simulink model "pfc"  (R2025b)
settings: Solver=VariableStepAuto  StartTime=0.0  StopTime=5  RelTol=1e-3
undefined symbols (not defined in the file): alpha, DiscIntNeverNeededParam, Ilimit, Izcd, K_Ton_max, Kff, Ki, Kp, Ncycle_min, Ton_max, Ton_min, Ton_startup_max, Ts_ctrl, Ts_v, Tstart, Vin_ff_max, Vin_ff_min, Vovp, Vref
libraries: fl_lib x29, nesl_utility x22, simulink x16, ee_lib x7, eeGeneralControl x4
settings Model: Creator=nickj  LastModifiedBy=nickj
settings DataIOCC: SignalLogging=off  DSMLogging=off  ReturnWorkspaceOutputs=off  LoggingIntervals=[4.8, 5]

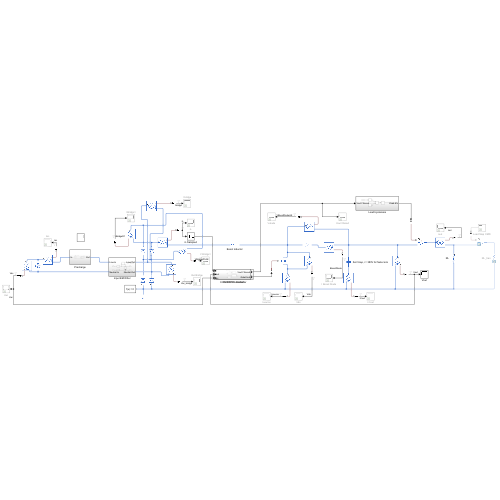
[thumbnail: Simulink's stored preview of the top-level diagram]
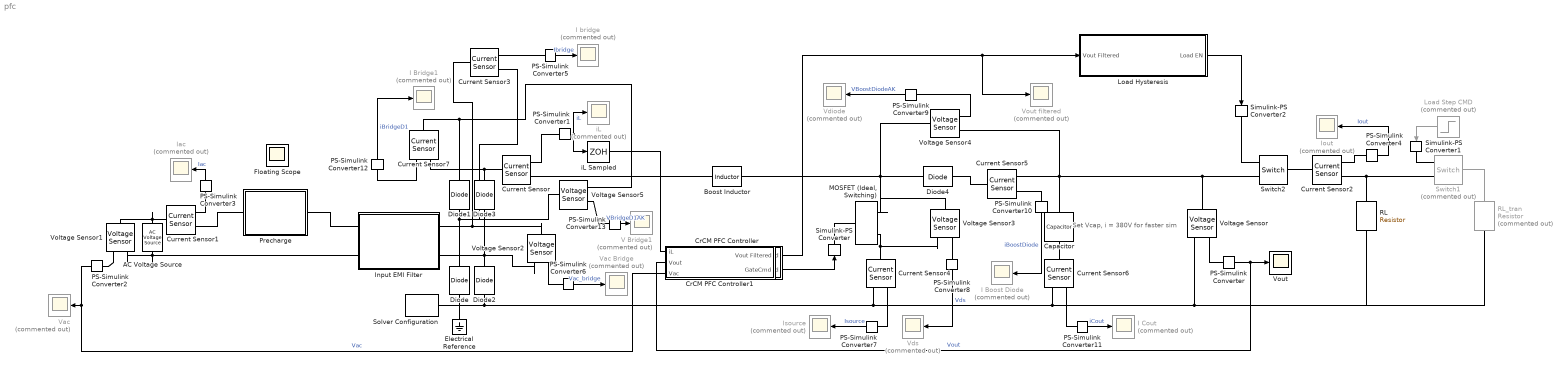
== system pfc ==
  note: Set Vcap, i = 380V for faster sim
  AC Voltage Source : fl_lib/Electrical/Electrical Sources/AC Voltage Source  amp=240*sqrt(2) V  shift=0 deg  frequency=60 Hz
  Boost Inductor : ee_lib/Passive/Inductor  l=270 uH  enable_L_tol=ee.enum.toleranceApplication.none  L_tol=20  tol_distribution=ee.enum.toleranceDistribution.uniform  nSigma=4  r=0.1 Ohm  g=1e-9 1/Ohm  enable_operating_limits=ee.enum.enable.no  operating_limit_action=ee.enum.passive.reportOpLim.warn  max_working_current=1 A  power_rating=1 W  i_L_specify=off  i_L_priority=High  i_L=0 A  i_L_nominal_specify=off  i_L_nominal_value=1  i_L_nominal_unit=A
  Capacitor : ee_lib/Passive/Capacitor  cap_option=ee.enum.passive.capacitor.capOption.const  c=220 uF  Cvec=[1e-05, 1e-06] F  Vvec=[0, 10] V  CV_table_symmetry=ee.enum.passive.capacitor.tableSymmetry.yes  f_vec=[1, 10] kHz  DFext_vec=[.8, 1.2]  enable_C_tol=ee.enum.toleranceApplication.none  averaging_period=0 s  C_tol=5  tol_distribution=ee.enum.toleranceDistribution.uniform  nSigma=4  r=0.3 Ohm  g=0 1/Ohm  enable_operating_limits=ee.enum.enable.no  operating_limit_action=ee.enum.passive.reportOpLim.warn  max_working_voltage_range=[-25, 25] V  power_rating=1 W  maxTemperature=85 degC  thermalEnable=false  thermalMass=1 J/K  i_specify=off  i_priority=None  i=0 A  i_nominal_specify=off  i_nominal_value=1  i_nominal_unit=A  v_specify=off  v_priority=None  v=380 V  v_nominal_specify=off  v_nominal_value=1  v_nominal_unit=V  vc_specify=off  vc_priority=High  vc=380 V  vc_nominal_specify=off  vc_nominal_value=1  vc_nominal_unit=V  T_specify=off  T_priority=None  T=298.15 K  T_nominal_specify=off  T_nominal_value=1  T_nominal_unit=K
  CrCM PFC Controller : Subsystem
  CrCM PFC Controller1 : Subsystem
  Current Sensor{,1..7} (8 alike) : fl_lib/Electrical/Electrical Sensors/Current Sensor
  Diode{,1..4} (5 alike) : fl_lib/Electrical/Electrical Elements/Diode  Vf=0.6 V  Ron=0.3 Ohm  Goff=1e-8 1/Ohm  i_specify=off  i_priority=None  i=0 A  i_nominal_specify=off  i_nominal_value=1  i_nominal_unit=A  v_specify=off  v_priority=None  v=0 V  v_nominal_specify=off  v_nominal_value=1  v_nominal_unit=V
  Electrical Reference : fl_lib/Electrical/Electrical Elements/Electrical Reference
  Floating Scope : Scope
      settings: IsFloating=on  Floating=on  ActiveDisplayString=4  Title=Gate CMD  ActiveDisplayYMinimum=-1.2499999999999998  ActiveDisplayYMaximum=11.25  DataLoggingVariableName=ScopeData33
  I Boost Diode : Scope  Commented=on
      settings: ActiveDisplayYMinimum=-50.843124756105674  ActiveDisplayYMaximum=457.58812280495118  DataLoggingVariableName=ScopeData24
  I Bridge1 : Scope  Commented=on
      settings: ActiveDisplayYMinimum=-7.204509005797358  ActiveDisplayYMaximum=47.078291389116806  DataLoggingVariableName=ScopeData26
  I Cout : Scope  Commented=on
      settings: ActiveDisplayYMinimum=-5.1833261982734609  ActiveDisplayYMaximum=46.649935784461157  DataLoggingVariableName=ScopeData25
  I bridge : Scope  Commented=on
      settings: ActiveDisplayYMinimum=-7.204509005797358  ActiveDisplayYMaximum=47.078291389116806  DataLoggingVariableName=ScopeData7
  Iac : Scope  Commented=on
      settings: ActiveDisplayYMinimum=-2.7208859223508548  ActiveDisplayYMaximum=2.8418563548590066  DataLoggingVariableName=ScopeData4
  Input EMI Filter : Subsystem
  Iout : Scope  Commented=on
      settings: ActiveDisplayYMinimum=-1.2771903163743626E-6  ActiveDisplayYMaximum=1.0183485230584859E-6  DataLoggingVariableName=ScopeData5
  Isource : Scope  Commented=on
      settings: ActiveDisplayYMinimum=-0.14948401946026615  ActiveDisplayYMaximum=1.3453561751423957  DataLoggingVariableName=ScopeData10
  Load Hysteresis : Subsystem
  Load Step CMD : Step  Commented=on  Time=2.5  Before=1  After=0  SampleTime=Ts_v
  "MOSFET (Ideal, Switching)" : ee_lib/Semiconductors & Converters/MOSFET (Ideal, Switching)  port_option=ee.enum.controlport.ps  Rds=0.3 Ohm  Goff=1e-8 1/Ohm  Vth=2 V  diode_param=ee.enum.semiconductors.protectionDiode.nodynamics  diode_Vf=0.8 V  diode_Ron=0.001 Ohm  diode_Goff=1e-5 1/Ohm  diode_C=50e-9 F  diode_iRM=-235 A  diode_iF=300 A  diode_idot=-50 A/us  diode_trr_param=ee.enum.converters.diodeReverseParam.trr_factor  diode_trr_factor=3  diode_trr=15 us  diode_Qrr=1500 s*uA  ids_specify=off  ids_priority=None  ids=0 A  ids_nominal_specify=off  ids_nominal_value=1  ids_nominal_unit=A  vds_specify=off  vds_priority=None  vds=0 V  vds_nominal_specify=off  vds_nominal_value=1  vds_nominal_unit=V  vgs_specify=off  vgs_priority=None  vgs=0 V  vgs_nominal_specify=off  vgs_nominal_value=1  vgs_nominal_unit=V  thermal_loss_option=ee.enum.converters.thermalLossOption.constantvalues  Von_data=[0, 1.8, 3.2, 6, 10, 16; 0, 2, 5.5, 9.5, 15, 25] V  Tj=[298.15, 448.15] K  Iout_data=[0, 20, 40, 60, 80, 100] A  Eon_data=[0, 55.04, 124.57, 235.53, 362.12; 0, 71.25, 161.25, 304.88, 468.75] * 1e-6 J  Eoff_data=[0, 18, 30, 56.1, 76.5; 0, 22.5, 37.5, 70.13, 95.63] * 1e-6 J  Eon_data_3D=[zeros(2, 5, 3)] J  Eoff_data_3D=[zeros(2, 5, 3)] J  Tj_loss=[298.15, 448.15] K  Iout_data_loss=[0, 10, 20, 30, 40] A  tabulateWithVds=false  Vds_loss=[0, 150, 300] V  Eon_scalar=22.86e-3 J  Eoff_scalar=17.14e-3 J  Voff=300 V  Iout_scalar=600 A  useCurrentFromPreviousCycle=false  useVoltageFromPreviousCycle=false  diodeModelType=ee.enum.converters.diodeModelType.pwl  diodeTableType=ee.enum.diode.tableType.IfMat  diode_ReverseIVType=ee.enum.diode.diodeReverseIV.constant  diode_IfMat=[.07, .12, .19, 1.75, 4.24, 7.32, 11.2; .16, .3, .72, 2.14, 4.02, 6.35, 9.12] A  diode_VfMat=[.9, 1.15, 1.25, 1.5, 1.75, 2.17, 2.6, 2.85; .58, .68, .75, 1.1, 1.38, 1.77, 2.27, 2.7] V  diode_TjVec=[25, 125] degC  diode_VfVec=[.5, .7, .9, 1.3, 1.7, 2.1, 2.5] V  diode_IfVec=[.1, .2, .5, 1, 2, 4, 7, 10] A  diode_IrMat=[1e-06, 2e-06, 5e-06, 1e-05, 2.5e-05, 5e-05, .0001; 2e-06, 5e-06, 1e-05, 4e-05, 8e-05, .0002, .0005] A  diode_VrMat=[10, 100, 200, 250, 300, 325, 350; 10, 70, 160, 220, 270, 300, 320] V  diode_VrVec=[10, 20, 40, 50, 70, 80, 100] V  diode_IrVec=[1e-06, 2e-06, 5e-06, 1e-05, 2e-05, 5e-05, .0001] A  diode_Vr=-600 V  diode_Ls=150 nH  diode_Erec=0.03 J  diode_rec_loss_model=ee.enum.diode.reverseRecoveryModel.fixed  diode_ErecVal=0 J  diode_scaleWithIandV=true  diode_ErecMat=zeros(2, 3) J  diode_TjrecVec=[298.15, 398.15] K  diode_IfrecVec=[.1, 1, 10] A  diode_IrecVal=10 A  diode_VrecVal=10 V  diode_tFilter=1 / 1000 / 100 s  separateThermalPortForDiode=false  thermal_network_parameterization=ee.enum.thermalNetworkTopology.external  Rth=[.03, .2] K/W  Rth_Cauer=[.03, .1, .2] K/W  Rth_Foster=[.08, .14, .22, .16] K/W  thermal_mass_parameterization=ee.enum.thermalNetwork.timeconstant  thermal_mass=[3, 25] J/K  thermal_mass_Cauer=[3, 10, 25] J/K  thermal_mass_Foster=[.001, .005, .05, .5] J/K  thermal_time_constant=[.1, 5] s  thermal_time_constant_Cauer=[.1, 1, 5] s  thermal_time_constant_Foster=[7e-05, .0007, .01, .08] s  thermal_mass_initial_temperatures=[25, 25] degC  thermal_mass_initial_temperatures_Cauer=[25, 25, 25] degC  junction_thermal_mass=0.1 J/K  Tvec_initial_Foster=[25, 25, 25, 25] degC  RthDiode=[.03, .2] K/W  RthCauerDiode=[.03, .1, .2] K/W  RthFosterDiode=[.03, .2] K/W  thermalMassDiode=[3, 25] J/K  thermalMassCauerDiode=[3, 10, 25] J/K  thermalMassFosterDiode=[33, 50] J/K  thermalTauDiode=[.1, 5] s  thermalTauCauerDiode=[.1, 1, 5] s  thermalTauFosterDiode=[1, 10] s  thermalMassInitTempDiode=[25, 25] degC  thermalMassInitTempCauerDiode=[25, 25, 25] degC  junctionthermalMassDiode=0.1 J/K  TVecInitialFosterDiode=[25, 25, 25, 25] degC  no_thermal_network=0  mosfet_junction_temperature_specify=off  mosfet_junction_temperature_priority=None  mosfet_junction_temperature=25 degC  mosfet_junction_temperature_nominal_specify=off  mosfet_junction_temperature_nominal_value=1  mosfet_junction_temperature_nominal_unit=degC  diode_junction_temperature_specify=off  diode_junction_temperature_priority=None  diode_junction_temperature=25 degC  diode_junction_temperature_nominal_specify=off  diode_junction_temperature_nominal_value=1  diode_junction_temperature_nominal_unit=degC  Qj_specify=off  Qj_priority=None  Qj=0 W  Qj_nominal_specify=off  Qj_nominal_value=1  Qj_nominal_unit=W  accumulatedSwitchingLosses_specify=off  accumulatedSwitchingLosses_priority=None  accumulatedSwitchingLosses=0 J
  PS-Simulink Converter{,1..13} (14 alike) : nesl_utility/PS-Simulink Converter  PhysicalDomain=network_engine_domain  SubClassName=ps_output  LeftPortType=input  RightPortType=output  PseudoPeriodic=off  Frequencies=[]  VectorFormat=inherit  Unit=inherit  AffineConversion=off
  Precharge : Subsystem
  RL : ee_lib/Passive/Resistor  R=8000 Ohm  enable_R_tol=ee.enum.toleranceApplication.none  R_tol=5  tol_distribution=ee.enum.toleranceDistribution.uniform  nSigma=4  enable_operating_limits=ee.enum.enable.no  operating_limit_action=ee.enum.passive.reportOpLim.warn  power_rating=1 W  max_working_voltage=100 V  noise_mode=ee.enum.sources.noise.Disabled  Tdevice=25 degC  sample_time=1e-3 s  repeatability=ee.enum.ic.repeatability.notRepeatable  user_seed=0  auto_seed=788174413  power_derating_T1=70 degC  power_derating_T2=155 degC  operating_temperature_range_vec=[-50, 150] degC  alpha=3.93e-3 1/K  Tmeas=25 degC  thermal_mass=100 J/K  temperature_specify=off  temperature_priority=High  temperature=298.15 K  temperature_nominal_specify=off  temperature_nominal_value=1  temperature_nominal_unit=K
  RL_tran : ee_lib/Passive/Resistor  Commented=on  R=2000 Ohm  enable_R_tol=ee.enum.toleranceApplication.none  R_tol=5  tol_distribution=ee.enum.toleranceDistribution.uniform  nSigma=4  enable_operating_limits=ee.enum.enable.no  operating_limit_action=ee.enum.passive.reportOpLim.warn  power_rating=1 W  max_working_voltage=100 V  noise_mode=ee.enum.sources.noise.Disabled  Tdevice=25 degC  sample_time=1e-3 s  repeatability=ee.enum.ic.repeatability.notRepeatable  user_seed=0  auto_seed=3499211588  power_derating_T1=70 degC  power_derating_T2=155 degC  operating_temperature_range_vec=[-50, 150] degC  alpha=3.93e-3 1/K  Tmeas=25 degC  thermal_mass=100 J/K  temperature_specify=off  temperature_priority=High  temperature=298.15 K  temperature_nominal_specify=off  temperature_nominal_value=1  temperature_nominal_unit=K
  Simulink-PS Converter : nesl_utility/Simulink-PS Converter  PhysicalDomain=network_engine_domain  SubClassName=ps_input  LeftPortType=input  RightPortType=output  PseudoPeriodic=off  Frequencies=[]  NoiseDistribution=none  NoiseParameters=[]  Unit=V  AffineConversion=off  FilteringAndDerivatives=zero  SimscapeFilterOrder=1  InputFilterTimeConstant=0.001  UdotUserProvided=0
  Simulink-PS Converter1 : nesl_utility/Simulink-PS Converter  PhysicalDomain=network_engine_domain  SubClassName=ps_input  LeftPortType=input  RightPortType=output  PseudoPeriodic=off  Frequencies=[]  NoiseDistribution=none  NoiseParameters=[]  Unit=1  AffineConversion=off  FilteringAndDerivatives=provide  SimscapeFilterOrder=1  InputFilterTimeConstant=0.001  UdotUserProvided=0
  Simulink-PS Converter2 : nesl_utility/Simulink-PS Converter  PhysicalDomain=network_engine_domain  SubClassName=ps_input  LeftPortType=input  RightPortType=output  PseudoPeriodic=off  Frequencies=[]  NoiseDistribution=none  NoiseParameters=[]  Unit=1  AffineConversion=off  FilteringAndDerivatives=provide  SimscapeFilterOrder=1  InputFilterTimeConstant=0.001  UdotUserProvided=0
  Solver Configuration : nesl_utility/Solver Configuration  PhysicalDomain=network_engine_domain  SubClassName=solver  LeftPortType=input  RightPortType=generic  Tones=[]  Harmonics=[]  SimulateNoise=off  Profile=off  UseLocalSampling=off  EnableSwitchedLinearOptims=on  FrequencyDomain=off  UseCCode=off  RelTol=0.001  AbsTol=0.001  MinStep=1e-09  ToWorkspace=off  RevertToSquareIcSolve=off  NumHomotopyIterations=100  PhasorMode=off  PhasorModeNumHarmonics=1  ConsistencySolver=NEWTON_XTOL_AFTER_FTOL  IndexReductionMethod=DerivativeReplacement  DoDC=off  ResidualTolerance=1e-09  ConsistencyTolSource=GLOBAL  ConsistencyAbsTol=0.001  ConsistencyRelTol=0.001  ConsistencyTolFactor=0.001  UseLocalSolver=off  LocalSolverChoice=NE_BACKWARD_EULER_ADVANCER  ResolveIndetEquations=on  FunctionEvalNumThread=1  LocalSolverSampleTime=0.001  DoFixedCost=off  MaxNonlinIter=3  MaxModeIter=2  ComputeImpulses=off  ImpulseIterations=2  LinearAlgebra=auto  LinearAlgebraNumThread=0  EquationFormulation=NE_TIME_EF  DelaysMemoryBudget=1024  AutomaticFiltering=on  FilteringTimeConstant=0.001  PartitionStorageMethod=AS_NEEDED  PartitionMemoryBudget=1024  PartitionMethod=ROBUST  MultibodyUseLocalSolver=off  MultibodyLocalSolverChoice=ODE1  MultibodyLocalSolverSampleTime=0.001
  Switch1 : fl_lib/Electrical/Electrical Elements/Switch  Commented=on  R_closed=0.01 Ohm  G_open=1e-8 1/Ohm  Threshold=0.5  i_specify=off  i_priority=None  i=0 A  i_nominal_specify=off  i_nominal_value=1  i_nominal_unit=A  v_specify=off  v_priority=None  v=0 V  v_nominal_specify=off  v_nominal_value=1  v_nominal_unit=V
  Switch2 : fl_lib/Electrical/Electrical Elements/Switch  R_closed=0.01 Ohm  G_open=1e-8 1/Ohm  Threshold=0.5  i_specify=off  i_priority=None  i=0 A  i_nominal_specify=off  i_nominal_value=1  i_nominal_unit=A  v_specify=off  v_priority=None  v=0 V  v_nominal_specify=off  v_nominal_value=1  v_nominal_unit=V
  V Bridge1 : Scope  Commented=on
      settings: ActiveDisplayYMinimum=-550.974255336967  ActiveDisplayYMaximum=568.62873247394509  DataLoggingVariableName=ScopeData27
  Vac : Scope  Commented=on
      settings: ActiveDisplayYMinimum=-261.34073882717638  ActiveDisplayYMaximum=282.8769482476535  DataLoggingVariableName=ScopeData2
  Vac Bridge : Scope  Commented=on
      settings: ActiveDisplayYMinimum=-550.974255336967  ActiveDisplayYMaximum=568.62873247394509  DataLoggingVariableName=ScopeData9
  Vdiode : Scope  Commented=on
      settings: ActiveDisplayYMinimum=-51.275619546528524  ActiveDisplayYMaximum=461.48057591875687  DataLoggingMaxPoints=1000  DataLoggingVariableName=ScopeData21
  Vds : Scope  Commented=on
      settings: ActiveDisplayYMinimum=-51.275619546528524  ActiveDisplayYMaximum=461.48057591875687  DataLoggingMaxPoints=1000  DataLoggingVariableName=ScopeData20
  Voltage Sensor{,1..5} (6 alike) : fl_lib/Electrical/Electrical Sensors/Voltage Sensor
  Vout : Scope
      settings: ActiveDisplayYMinimum=397.4742246444398  ActiveDisplayYMaximum=403.09007676849239  DataLoggingMaxPoints=1000
  Vout filtered : Scope  Commented=on
      settings: ActiveDisplayYMinimum=-1  ActiveDisplayYMaximum=1  DataLoggingVariableName=ScopeData18
  iL : Scope  Commented=on
      settings: ActiveDisplayYMinimum=-0.53899778989622149  ActiveDisplayYMaximum=4.8509800679226229
  iL Sampled : ZeroOrderHold  SampleTime=Ts_ctrl
  wires:
  PS-Simulink Converter1/1 -> iL Sampled/1, iL/1  "iL"
  PS-Simulink Converter/1 -> Vout/1, CrCM PFC Controller/2(Vout)  "Vout"
  PS-Simulink Converter2/1 -> CrCM PFC Controller/3(Vac), Vac/1  "Vac"
  CrCM PFC Controller/2(GateCmd) -> Simulink-PS Converter/1
  iL Sampled/1 -> CrCM PFC Controller/1(iL)
  PS-Simulink Converter3/1 -> Iac/1  "Iac"
  PS-Simulink Converter4/1 -> Iout/1  "Iout"
  PS-Simulink Converter5/1 -> I bridge/1  "Ibridge"
  PS-Simulink Converter6/1 -> Vac Bridge/1  "Vac_bridge"
  PS-Simulink Converter7/1 -> Isource/1  "Isource"
  CrCM PFC Controller/1(Vout Filtered) -> Load Hysteresis/1(Vout Filtered), Vout filtered/1
  PS-Simulink Converter8/1 -> Vds/1  "Vds"
  PS-Simulink Converter9/1 -> Vdiode/1  "VBoostDiodeAK"
  Load Hysteresis/1(Load EN) -> Simulink-PS Converter2/1
  PS-Simulink Converter10/1 -> I Boost Diode/1  "iBoostDiode"
  PS-Simulink Converter11/1 -> I Cout/1  "iCout"
  PS-Simulink Converter12/1 -> I Bridge1/1  "iBridgeD1"
  PS-Simulink Converter13/1 -> V Bridge1/1  "VBridgeD1AK"
  Load Step CMD/1 -> Simulink-PS Converter1/1
  connections:
  RL/RConn1 -- RL_tran/RConn1 -- Voltage Sensor/RConn2 -- Current Sensor6/RConn2 -- Current Sensor4/RConn2 -- Diode/LConn1 -- Electrical Reference/LConn1 -- Solver Configuration/RConn1 -- Diode2/LConn1
  Current Sensor/LConn1 -- Current Sensor7/RConn2 -- Diode3/RConn1
  Diode/RConn1 -- Voltage Sensor5/LConn1 -- Current Sensor3/RConn2 -- Diode1/LConn1
  Current Sensor/RConn1 -- PS-Simulink Converter1/LConn1
  Voltage Sensor4/LConn1 -- Boost Inductor/RConn1 -- Voltage Sensor3/LConn1 -- "MOSFET (Ideal, Switching)"/RConn1 -- Diode4/LConn1
  Voltage Sensor/LConn1 -- Switch2/RConn2 -- Current Sensor5/RConn2 -- Voltage Sensor4/RConn2 -- Capacitor/LConn1
  Current Sensor/RConn2 -- Boost Inductor/LConn1
  Voltage Sensor/RConn1 -- PS-Simulink Converter/LConn1
  Voltage Sensor1/RConn1 -- PS-Simulink Converter2/LConn1
  Simulink-PS Converter/RConn1 -- "MOSFET (Ideal, Switching)"/LConn1
  AC Voltage Source/LConn1 -- Current Sensor1/LConn1 -- Voltage Sensor1/LConn1
  Current Sensor1/RConn1 -- PS-Simulink Converter3/LConn1
  Current Sensor2/RConn2 -- Switch1/RConn2 -- RL/LConn1
  Current Sensor2/RConn1 -- PS-Simulink Converter4/LConn1
  Diode2/RConn1 -- Input EMI Filter/RConn2 -- Voltage Sensor2/RConn2 -- Diode3/LConn1
  Voltage Sensor1/RConn2 -- AC Voltage Source/RConn1 -- Input EMI Filter/LConn2
  Current Sensor3/LConn1 -- Voltage Sensor2/LConn1 -- Input EMI Filter/RConn1
  Current Sensor3/RConn1 -- PS-Simulink Converter5/LConn1
  PS-Simulink Converter6/LConn1 -- Voltage Sensor2/RConn1
  Current Sensor4/LConn1 -- Voltage Sensor3/RConn2 -- "MOSFET (Ideal, Switching)"/RConn2
  PS-Simulink Converter7/LConn1 -- Current Sensor4/RConn1
  Simulink-PS Converter2/RConn1 -- Switch2/RConn1
  Switch2/LConn1 -- Current Sensor2/LConn1
  Voltage Sensor3/RConn1 -- PS-Simulink Converter8/LConn1
  PS-Simulink Converter9/LConn1 -- Voltage Sensor4/RConn1
  Precharge/LConn1 -- Current Sensor1/RConn2
  Precharge/RConn1 -- Input EMI Filter/LConn1
  Current Sensor5/LConn1 -- Diode4/RConn1
  PS-Simulink Converter10/LConn1 -- Current Sensor5/RConn1
  Current Sensor6/LConn1 -- Capacitor/RConn1
  PS-Simulink Converter11/LConn1 -- Current Sensor6/RConn1
  Current Sensor7/LConn1 -- Voltage Sensor5/RConn2 -- Diode1/RConn1
  Current Sensor7/RConn1 -- PS-Simulink Converter12/LConn1
  PS-Simulink Converter13/LConn1 -- Voltage Sensor5/RConn1
  Switch1/LConn1 -- RL_tran/LConn1
  Simulink-PS Converter1/RConn1 -- Switch1/RConn1

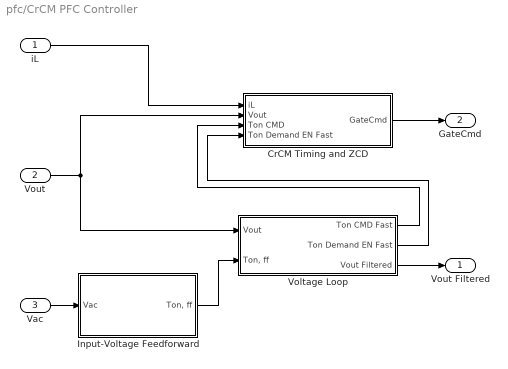
== system pfc/CrCM PFC Controller ==
  iL : Inport
  Vout : Inport  Port=2
  Vac : Inport  Port=3
  CrCM Timing and ZCD : Subsystem
  Input-Voltage Feedforward : Subsystem
  Voltage Loop : Subsystem
  Vout Filtered : Outport
  GateCmd : Outport  Port=2
  wires:
  iL/1 -> CrCM Timing and ZCD/1(iL)
  Vout/1 -> Voltage Loop/1(Vout), CrCM Timing and ZCD/2(Vout)
  CrCM Timing and ZCD/1(GateCmd) -> GateCmd/1
  Voltage Loop/1(Ton CMD Fast) -> CrCM Timing and ZCD/3(Ton CMD)
  Vac/1 -> Input-Voltage Feedforward/1(Vac)
  Input-Voltage Feedforward/1("Ton, ff") -> Voltage Loop/2("Ton, ff")
  Voltage Loop/3(Vout Filtered) -> Vout Filtered/1
  Voltage Loop/2(Ton Demand EN Fast) -> CrCM Timing and ZCD/4(Ton Demand EN Fast)

== system pfc/CrCM PFC Controller1 ==
  iL : Inport
  Vout : Inport  Port=2
  Vac : Inport  Port=3
  CrCM Timing and ZCD : Subsystem
  Input-Voltage Feedforward : Subsystem
  Voltage Loop : Subsystem
  Vout Filtered : Outport
  GateCmd : Outport  Port=2
  wires:
  Voltage Loop/2(Ton Demand EN Fast) -> CrCM Timing and ZCD/4(Ton Demand EN Fast)
  Voltage Loop/3(Vout Filtered) -> Vout Filtered/1
  Input-Voltage Feedforward/1("Ton, ff") -> Voltage Loop/2("Ton, ff")
  Vac/1 -> Input-Voltage Feedforward/1(Vac)
  Voltage Loop/1(Ton CMD Fast) -> CrCM Timing and ZCD/3(Ton CMD)
  CrCM Timing and ZCD/1(GateCmd) -> GateCmd/1
  Vout/1 -> CrCM Timing and ZCD/2(Vout), Voltage Loop/1(Vout)
  iL/1 -> CrCM Timing and ZCD/1(iL)

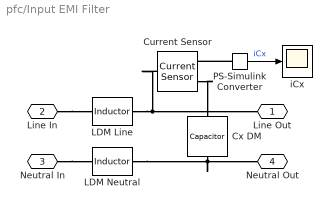
== system pfc/Input EMI Filter ==
  Current Sensor : fl_lib/Electrical/Electrical Sensors/Current Sensor
  Cx DM : fl_lib/Electrical/Electrical Elements/Capacitor  c=100 nF  r=0.2 Ohm  g=0 1/Ohm  i_specify=off  i_priority=None  i=0 A  i_nominal_specify=off  i_nominal_value=1  i_nominal_unit=A  v_specify=off  v_priority=None  v=0 V  v_nominal_specify=off  v_nominal_value=1  v_nominal_unit=V  vc_specify=off  vc_priority=High  vc=0 V  vc_nominal_specify=off  vc_nominal_value=1  vc_nominal_unit=V
  LDM Line : ee_lib/Passive/Inductor  l=1 mH  enable_L_tol=ee.enum.toleranceApplication.none  L_tol=20  tol_distribution=ee.enum.toleranceDistribution.uniform  nSigma=4  r=0.05 Ohm  g=1e-9 1/Ohm  enable_operating_limits=ee.enum.enable.no  operating_limit_action=ee.enum.passive.reportOpLim.warn  max_working_current=1 A  power_rating=1 W  i_L_specify=off  i_L_priority=High  i_L=0 A  i_L_nominal_specify=off  i_L_nominal_value=1  i_L_nominal_unit=A
  LDM Neutral : ee_lib/Passive/Inductor  l=1 mH  enable_L_tol=ee.enum.toleranceApplication.none  L_tol=20  tol_distribution=ee.enum.toleranceDistribution.uniform  nSigma=4  r=0.05 Ohm  g=1e-9 1/Ohm  enable_operating_limits=ee.enum.enable.no  operating_limit_action=ee.enum.passive.reportOpLim.warn  max_working_current=1 A  power_rating=1 W  i_L_specify=off  i_L_priority=High  i_L=0 A  i_L_nominal_specify=off  i_L_nominal_value=1  i_L_nominal_unit=A
  PS-Simulink Converter : nesl_utility/PS-Simulink Converter  PhysicalDomain=network_engine_domain  SubClassName=ps_output  LeftPortType=input  RightPortType=output  PseudoPeriodic=off  Frequencies=[]  VectorFormat=inherit  Unit=inherit  AffineConversion=off
  iCx : Scope
      settings: DataLoggingVariableName=ScopeData23
  Line Out : PMIOPort  Side=Right
  Line In : PMIOPort  Port=2  Side=Left
  Neutral In : PMIOPort  Port=3  Side=Left
  Neutral Out : PMIOPort  Port=4  Side=Right
  wires:
  PS-Simulink Converter/1 -> iCx/1  "iCx"
  connections:
  Cx DM/RConn1 -- Neutral Out/RConn1 -- LDM Neutral/RConn1
  LDM Line/RConn1 -- Line Out/RConn1 -- Current Sensor/LConn1
  Neutral In/RConn1 -- LDM Neutral/LConn1
  Line In/RConn1 -- LDM Line/LConn1
  Current Sensor/RConn2 -- Cx DM/LConn1
  PS-Simulink Converter/LConn1 -- Current Sensor/RConn1

== system pfc/Load Hysteresis ==
  Vout Filtered : Inport
  Load Arm : Step  Time=0.212  SampleTime=0
  Load CMD : Product
  Load READY : Relay  OnSwitchValue=370  OffSwitchValue=340
  Unit Delay : UnitDelay  SampleTime=Ts_v  HasFrameUpgradeWarning=on
  Load EN : Outport
  wires:
  Load Arm/1 -> Load CMD/2
  Load READY/1 -> Load CMD/1
  Unit Delay/1 -> Load EN/1  "LoadCmd"
  Load CMD/1 -> Unit Delay/1
  Vout Filtered/1 -> Load READY/1

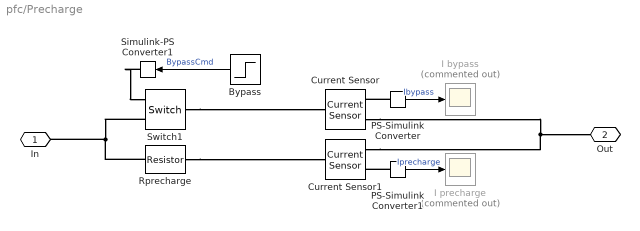
== system pfc/Precharge ==
  Bypass : Step  Time=0.2  SampleTime=0
  Current Sensor : fl_lib/Electrical/Electrical Sensors/Current Sensor
  Current Sensor1 : fl_lib/Electrical/Electrical Sensors/Current Sensor
  I bypass : Scope  Commented=on
      settings: DataLoggingVariableName=ScopeData22
  I precharge : Scope  Commented=on
      settings: DataLoggingVariableName=ScopeData19
  PS-Simulink Converter : nesl_utility/PS-Simulink Converter  PhysicalDomain=network_engine_domain  SubClassName=ps_output  LeftPortType=input  RightPortType=output  PseudoPeriodic=off  Frequencies=[]  VectorFormat=inherit  Unit=inherit  AffineConversion=off
  PS-Simulink Converter1 : nesl_utility/PS-Simulink Converter  PhysicalDomain=network_engine_domain  SubClassName=ps_output  LeftPortType=input  RightPortType=output  PseudoPeriodic=off  Frequencies=[]  VectorFormat=inherit  Unit=inherit  AffineConversion=off
  Rprecharge : fl_lib/Electrical/Electrical Elements/Resistor  R=82 Ohm  i_specify=off  i_priority=None  i=0 A  i_nominal_specify=off  i_nominal_value=1  i_nominal_unit=A  v_specify=off  v_priority=None  v=0 V  v_nominal_specify=off  v_nominal_value=1  v_nominal_unit=V
  Simulink-PS Converter1 : nesl_utility/Simulink-PS Converter  PhysicalDomain=network_engine_domain  SubClassName=ps_input  LeftPortType=input  RightPortType=output  PseudoPeriodic=off  Frequencies=[]  NoiseDistribution=none  NoiseParameters=[]  Unit=1  AffineConversion=off  FilteringAndDerivatives=provide  SimscapeFilterOrder=1  InputFilterTimeConstant=0.001  UdotUserProvided=0
  Switch1 : fl_lib/Electrical/Electrical Elements/Switch  R_closed=0.01 Ohm  G_open=1e-8 1/Ohm  Threshold=0.5  i_specify=off  i_priority=None  i=0 A  i_nominal_specify=off  i_nominal_value=1  i_nominal_unit=A  v_specify=off  v_priority=None  v=0 V  v_nominal_specify=off  v_nominal_value=1  v_nominal_unit=V
  In : PMIOPort  Side=Left
  Out : PMIOPort  Port=2  Side=Right
  wires:
  Bypass/1 -> Simulink-PS Converter1/1  "BypassCmd"
  PS-Simulink Converter1/1 -> I precharge/1  "Iprecharge"
  PS-Simulink Converter/1 -> I bypass/1  "Ibypass"
  connections:
  Rprecharge/LConn1 -- In/RConn1 -- Switch1/RConn2
  Simulink-PS Converter1/RConn1 -- Switch1/RConn1
  Switch1/LConn1 -- Current Sensor/LConn1
  Current Sensor/RConn2 -- Current Sensor1/RConn2 -- Out/RConn1
  Rprecharge/RConn1 -- Current Sensor1/LConn1
  PS-Simulink Converter/LConn1 -- Current Sensor/RConn1
  PS-Simulink Converter1/LConn1 -- Current Sensor1/RConn1

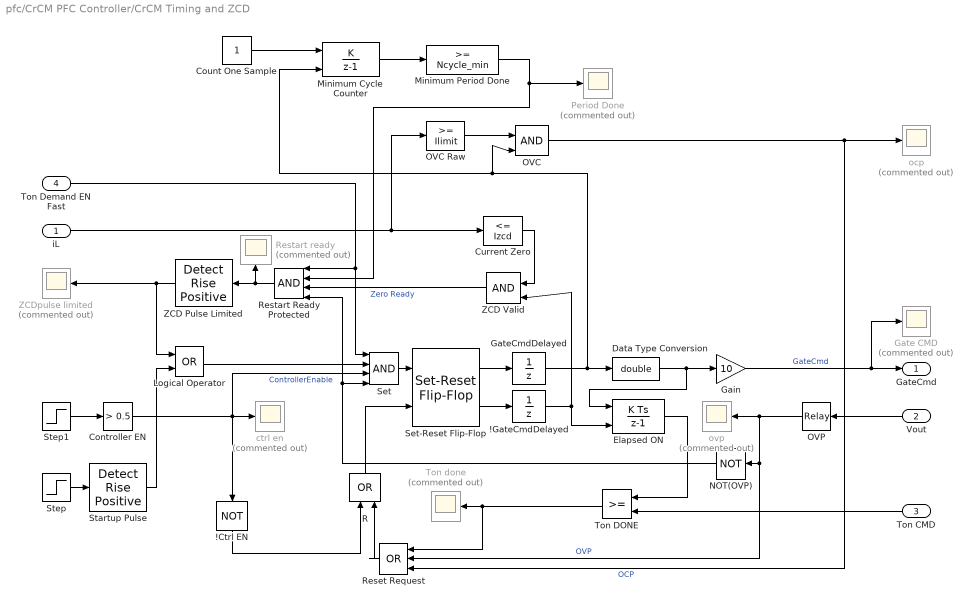
== system pfc/CrCM PFC Controller/CrCM Timing and ZCD ==
  iL : Inport
  Vout : Inport  Port=2
  Ton CMD : Inport  Port=3
  Ton Demand EN Fast : Inport  Port=4
  !Ctrl EN : Logic  Operator=NOT  IconShape=distinctive  AllPortsSameDT=off  OutDataTypeStr=boolean
  !GateCmdDelayed : UnitDelay  SampleTime=Ts_ctrl  HasFrameUpgradeWarning=on
  Controller EN : simulink/Logic and Bit Operations/Compare To Constant  relop=>  const=0.5  OutDataTypeStr=boolean
  Count One Sample : Constant  SampleTime=Ts_ctrl
  Current Zero : simulink/Logic and Bit Operations/Compare To Constant  relop=<=  const=Izcd  OutDataTypeStr=boolean
  Data Type Conversion : DataTypeConversion  OutDataTypeStr=double  SaturateOnIntegerOverflow=off  RndMeth=Floor
  Elapsed ON : DiscreteIntegrator  ExternalReset=level  SampleTime=Ts_ctrl  ICPrevOutput=DiscIntNeverNeededParam  ICPrevScaledInput=DiscIntNeverNeededParam
  Gain : Gain  Gain=10
  Gate CMD : Scope  Commented=on
      settings: ActiveDisplayYMinimum=-1.2895256916996045  ActiveDisplayYMaximum=11.210474308300396  DataLoggingVariableName=ScopeData11
  GateCmdDelayed : UnitDelay  SampleTime=Ts_ctrl  HasFrameUpgradeWarning=on
  Logical Operator : Logic  Operator=OR  AllPortsSameDT=off  OutDataTypeStr=boolean
  Minimum Cycle Counter : DiscreteIntegrator  IntegratorMethod=Accumulation: Forward Euler  ExternalReset=rising  SampleTime=Ts_ctrl  LimitOutput=on  UpperSaturationLimit=Ncycle_min  LowerSaturationLimit=0  ICPrevOutput=DiscIntNeverNeededParam  ICPrevScaledInput=DiscIntNeverNeededParam
  Minimum Period Done : simulink/Logic and Bit Operations/Compare To Constant  relop=>=  const=Ncycle_min  OutDataTypeStr=boolean
  NOT(OVP) : Logic  Operator=NOT  IconShape=distinctive  AllPortsSameDT=off  OutDataTypeStr=boolean
  OVC : Logic  IconShape=distinctive  AllPortsSameDT=off  OutDataTypeStr=boolean
  OVC Raw : simulink/Logic and Bit Operations/Compare To Constant  relop=>=  const=Ilimit  OutDataTypeStr=boolean
  OVP : Relay  OnSwitchValue=Vovp  OffSwitchValue=Vovp-10
  Period Done : Scope  Commented=on
      settings: ActiveDisplayYMinimum=-0.12499999999999997  ActiveDisplayYMaximum=1.125  DataLoggingVariableName=ScopeData28
  R : Logic  Operator=OR  IconShape=distinctive  AllPortsSameDT=off  OutDataTypeStr=boolean
  Reset Request : Logic  Operator=OR  Inputs=3  IconShape=distinctive  AllPortsSameDT=off  OutDataTypeStr=boolean
  Restart Ready Protected : Logic  Inputs=4  AllPortsSameDT=off  OutDataTypeStr=boolean
  Restart ready : Scope  Commented=on
      settings: ActiveDisplayYMinimum=-0.12180825947879081  ActiveDisplayYMaximum=1.1472265317427257  DataLoggingVariableName=ScopeData3
  Set : Logic  Inputs=4  AllPortsSameDT=off  OutDataTypeStr=boolean
  Set-Reset Flip-Flop : eeGeneralControl/Set-Reset Flip-Flop  LabelModeActiveChoice=Discrete  UndefState=Reset  Q0=0  Ts=Ts_ctrl
      settings: LibrarySourceBlock=ee_sl_lib/General Control/Set-Reset Flip-Flop
  Startup Pulse : simulink/Logic and Bit Operations/Detect Rise Positive  vinit=0  OutDataTypeStr=boolean
  Step : Step  Time=Tstart  SampleTime=Ts_ctrl
  Step1 : Step  Time=0.21  SampleTime=0
  Ton DONE : RelationalOperator  OutDataTypeStr=boolean  RndMeth=Simplest  InputSameDT=off
  Ton done : Scope  Commented=on
      settings: ActiveDisplayYMinimum=-0.12499999999999997  ActiveDisplayYMaximum=1.125  DataLoggingVariableName=ScopeData16
  ZCD Pulse Limited : simulink/Logic and Bit Operations/Detect Rise Positive  vinit=0  OutDataTypeStr=boolean
  ZCD Valid : Logic  IconShape=distinctive  AllPortsSameDT=off  OutDataTypeStr=boolean
  ZCDpulse limited : Scope  Commented=on
      settings: ActiveDisplayYMinimum=-0.12499999999999997  ActiveDisplayYMaximum=1.125  DataLoggingVariableName=ScopeData13
  ctrl en : Scope  Commented=on
      settings: ActiveDisplayYMinimum=-0.067572366136101847  ActiveDisplayYMaximum=1.141032196932009  DataLoggingVariableName=ScopeData17
  ocp : Scope  Commented=on
      settings: ActiveDisplayYMinimum=-1  ActiveDisplayYMaximum=1  DataLoggingVariableName=ScopeData15
  ovp : Scope  Commented=on
      settings: ActiveDisplayYMinimum=-1  ActiveDisplayYMaximum=1  DataLoggingVariableName=ScopeData14
  GateCmd : Outport
  wires:
  Startup Pulse/1 -> Logical Operator/2
  Step/1 -> Startup Pulse/1
  iL/1 -> Current Zero/1, OVC Raw/1
  Set-Reset Flip-Flop/1 -> GateCmdDelayed/1
  OVP/1 -> ovp/1, Reset Request/2, NOT(OVP)/1  "OVP"
  Current Zero/1 -> ZCD Valid/1
  ZCD Valid/1 -> Restart Ready Protected/3  "Zero Ready"
  OVC Raw/1 -> OVC/1
  OVC/1 -> Reset Request/3, ocp/1  "OCP"
  ZCD Pulse Limited/1 -> ZCDpulse limited/1, Logical Operator/1
  NOT(OVP)/1 -> Set/4, Restart Ready Protected/4
  Logical Operator/1 -> Set/2
  Data Type Conversion/1 -> Elapsed ON/1, Gain/1
  Vout/1 -> OVP/1
  Gain/1 -> Gate CMD/1, GateCmd/1  "GateCmd"
  Set-Reset Flip-Flop/2 -> !GateCmdDelayed/1
  !GateCmdDelayed/1 -> ZCD Valid/2, Elapsed ON/2
  Elapsed ON/1 -> Ton DONE/1
  Ton DONE/1 -> Ton done/1, Reset Request/1
  Ton CMD/1 -> Ton DONE/2
  Set/1 -> Set-Reset Flip-Flop/1
  Step1/1 -> Controller EN/1
  Controller EN/1 -> !Ctrl EN/1, ctrl en/1, Set/3  "ControllerEnable"
  R/1 -> Set-Reset Flip-Flop/2
  Reset Request/1 -> R/2
  !Ctrl EN/1 -> R/1
  Minimum Period Done/1 -> Restart Ready Protected/2, Period Done/1
  Minimum Cycle Counter/1 -> Minimum Period Done/1
  Count One Sample/1 -> Minimum Cycle Counter/1
  GateCmdDelayed/1 -> Minimum Cycle Counter/2, OVC/2, Data Type Conversion/1
  Restart Ready Protected/1 -> ZCD Pulse Limited/1, Restart ready/1
  Ton Demand EN Fast/1 -> Set/1, Restart Ready Protected/1

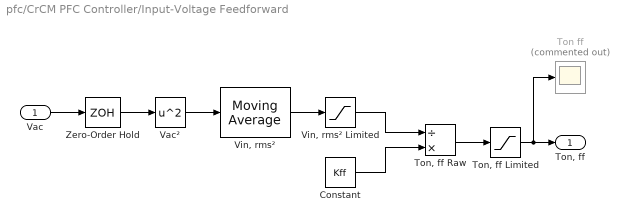
== system pfc/CrCM PFC Controller/Input-Voltage Feedforward ==
  Vac : Inport
  Constant : Constant  Value=Kff
  Ton ff : Scope  Commented=on
      settings: DataLoggingVariableName=ScopeData29
  "Ton, ff Limited" : Saturate  UpperLimit=Ton_max  LowerLimit=Ton_min
  "Ton, ff Raw" : Product  Inputs=/*
  Vac² : Math  Operator=square
  "Vin, rms²" : eeGeneralControl/Moving Average  VariantControl=Variant1  LabelModeActiveChoice=Discrete  f=Favg  x0=Vin_ff_max^2  BufferSize=8192  Ts=Ts_v
      settings: LibrarySourceBlock=ee_sl_lib/General Control/Moving Average
  "Vin, rms² Limited" : Saturate  UpperLimit=Vin_ff_max^2  LowerLimit=Vin_ff_min^2
  Zero-Order Hold : ZeroOrderHold  SampleTime=Ts_v
  "Ton, ff" : Outport
  wires:
  "Ton, ff Limited"/1 -> "Ton, ff"/1, Ton ff/1
  "Ton, ff Raw"/1 -> "Ton, ff Limited"/1
  Constant/1 -> "Ton, ff Raw"/2
  Vac/1 -> Zero-Order Hold/1
  Zero-Order Hold/1 -> Vac²/1
  Vac²/1 -> "Vin, rms²"/1
  "Vin, rms²"/1 -> "Vin, rms² Limited"/1
  "Vin, rms² Limited"/1 -> "Ton, ff Raw"/1

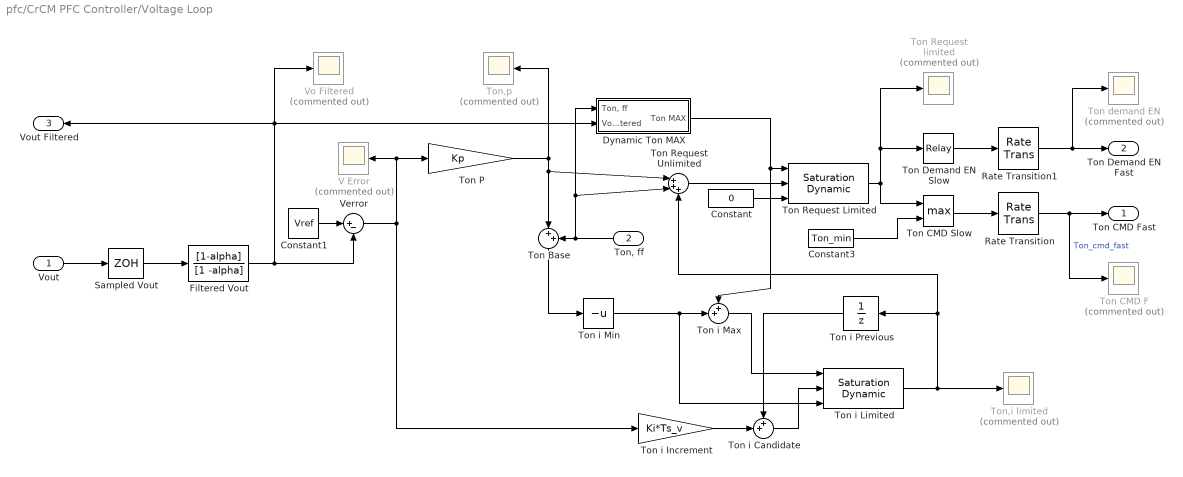
== system pfc/CrCM PFC Controller/Voltage Loop ==
  Vout : Inport
  "Ton, ff" : Inport  Port=2
  Constant : Constant  Value=0
  Constant1 : Constant  Value=Vref
  Constant3 : Constant  Value=Ton_min
  Dynamic Ton MAX : Subsystem
  Filtered Vout : DiscreteFilter  Numerator=[1-alpha]  Denominator=[1 -alpha]
  Rate Transition : RateTransition  OutPortSampleTime=Ts_ctrl
  Rate Transition1 : RateTransition  OutPortSampleTime=Ts_ctrl
  Sampled Vout : ZeroOrderHold  SampleTime=Ts_v
  Ton Base : Sum  Inputs=|++
  Ton CMD F : Scope  Commented=on
      settings: ActiveDisplayYMinimum=-6.2402343750000437E-7  ActiveDisplayYMaximum=5.61621093750004E-6  DataLoggingVariableName=ScopeData4
  Ton CMD Slow : MinMax  Function=max  Inputs=2
  Ton Demand EN Slow : Relay  OnSwitchValue=0.25e-6  OffSwitchValue=0.15e-6
  Ton P : Gain  Gain=Kp
  Ton Request Limited : simulink/Discontinuities/Saturation Dynamic  OutMin=[]  OutMax=[]  OutDataTypeStr=Inherit: Same as second input  OutDataType=fixdt(1, 16)  OutScaling=2^-10  DoSatur=off
  Ton Request Unlimited : Sum  Inputs=|+++
  Ton Request limited : Scope  Commented=on
      settings: ActiveDisplayYMinimum=-6.2402343750000437E-7  ActiveDisplayYMaximum=5.61621093750004E-6  DataLoggingVariableName=ScopeData31
  Ton demand EN : Scope  Commented=on
      settings: ActiveDisplayYMinimum=-0.12499999999999997  ActiveDisplayYMaximum=1.125  DataLoggingVariableName=ScopeData32
  Ton i Candidate : Sum  Inputs=++|
  Ton i Increment : Gain  Gain=Ki*Ts_v
  Ton i Limited : simulink/Discontinuities/Saturation Dynamic  OutMin=[]  OutMax=[]  OutDataTypeStr=Inherit: Same as second input  OutDataType=fixdt(1, 16)  OutScaling=2^-10  DoSatur=off
  Ton i Max : Sum  Inputs=++|
  Ton i Min : UnaryMinus
  Ton i Previous : UnitDelay  SampleTime=Ts_v  HasFrameUpgradeWarning=on
  Ton,i limited : Scope  Commented=on
      settings: ActiveDisplayYMinimum=-2.1964491979871354E-5  ActiveDisplayYMaximum=-4.8570738523942261E-7  DataLoggingVariableName=ScopeData5
  Ton,p : Scope  Commented=on
      settings: ActiveDisplayYMinimum=-1  ActiveDisplayYMaximum=1  DataLoggingVariableName=ScopeData6
  V Error : Scope  Commented=on
      settings: ActiveDisplayYMinimum=-54.436797901424178  ActiveDisplayYMaximum=450.4929775446027  DataLoggingVariableName=ScopeData12
  Verror : Sum  Inputs=|+-
  Vo Filtered : Scope  Commented=on
      settings: ActiveDisplayYMinimum=-52.339947093671832  ActiveDisplayYMaximum=471.05952384304663  DataLoggingVariableName=ScopeData30
  Ton CMD Fast : Outport
  Ton Demand EN Fast : Outport  Port=2
  Vout Filtered : Outport  Port=3
  wires:
  Filtered Vout/1 -> Verror/2, Dynamic Ton MAX/2(Vout Filtered), Vo Filtered/1, Vout Filtered/1
  Verror/1 -> V Error/1, Ton P/1, Ton i Increment/1
  Ton Request Unlimited/1 -> Ton Request Limited/2
  Rate Transition/1 -> Ton CMD Fast/1, Ton CMD F/1  "Ton_cmd_fast"
  Sampled Vout/1 -> Filtered Vout/1
  Constant1/1 -> Verror/1
  Ton P/1 -> Ton Base/1, Ton Request Unlimited/1, Ton,p/1
  Vout/1 -> Sampled Vout/1
  "Ton, ff"/1 -> Ton Base/2, Dynamic Ton MAX/1("Ton, ff"), Ton Request Unlimited/2
  Constant/1 -> Ton Request Limited/3
  Dynamic Ton MAX/1(Ton MAX) -> Ton i Max/1, Ton Request Limited/1
  Ton Base/1 -> Ton i Min/1
  Ton i Max/1 -> Ton i Limited/1
  Ton i Min/1 -> Ton i Max/2, Ton i Limited/3
  Ton i Candidate/1 -> Ton i Limited/2
  Ton i Limited/1 -> Ton,i limited/1, Ton i Previous/1, Ton Request Unlimited/3
  Ton i Previous/1 -> Ton i Candidate/1
  Ton i Increment/1 -> Ton i Candidate/2
  Ton Request Limited/1 -> Ton Request limited/1, Ton Demand EN Slow/1, Ton CMD Slow/1
  Constant3/1 -> Ton CMD Slow/2
  Ton CMD Slow/1 -> Rate Transition/1
  Ton Demand EN Slow/1 -> Rate Transition1/1
  Rate Transition1/1 -> Ton demand EN/1, Ton Demand EN Fast/1

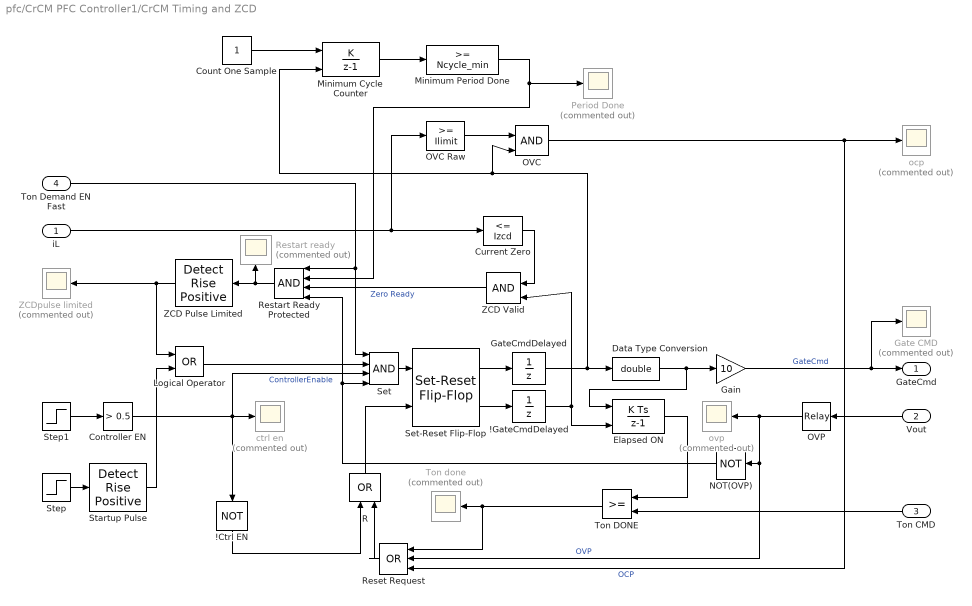
== system pfc/CrCM PFC Controller1/CrCM Timing and ZCD ==
  iL : Inport
  Vout : Inport  Port=2
  Ton CMD : Inport  Port=3
  Ton Demand EN Fast : Inport  Port=4
  !Ctrl EN : Logic  Operator=NOT  IconShape=distinctive  AllPortsSameDT=off  OutDataTypeStr=boolean
  !GateCmdDelayed : UnitDelay  SampleTime=Ts_ctrl  HasFrameUpgradeWarning=on
  Controller EN : simulink/Logic and Bit Operations/Compare To Constant  relop=>  const=0.5  OutDataTypeStr=boolean
  Count One Sample : Constant  SampleTime=Ts_ctrl
  Current Zero : simulink/Logic and Bit Operations/Compare To Constant  relop=<=  const=Izcd  OutDataTypeStr=boolean
  Data Type Conversion : DataTypeConversion  OutDataTypeStr=double  SaturateOnIntegerOverflow=off  RndMeth=Floor
  Elapsed ON : DiscreteIntegrator  ExternalReset=level  SampleTime=Ts_ctrl  ICPrevOutput=DiscIntNeverNeededParam  ICPrevScaledInput=DiscIntNeverNeededParam
  Gain : Gain  Gain=10
  Gate CMD : Scope  Commented=on
      settings: ActiveDisplayYMinimum=-1.2895256916996045  ActiveDisplayYMaximum=11.210474308300396  DataLoggingVariableName=ScopeData11
  GateCmdDelayed : UnitDelay  SampleTime=Ts_ctrl  HasFrameUpgradeWarning=on
  Logical Operator : Logic  Operator=OR  AllPortsSameDT=off  OutDataTypeStr=boolean
  Minimum Cycle Counter : DiscreteIntegrator  IntegratorMethod=Accumulation: Forward Euler  ExternalReset=rising  SampleTime=Ts_ctrl  LimitOutput=on  UpperSaturationLimit=Ncycle_min  LowerSaturationLimit=0  ICPrevOutput=DiscIntNeverNeededParam  ICPrevScaledInput=DiscIntNeverNeededParam
  Minimum Period Done : simulink/Logic and Bit Operations/Compare To Constant  relop=>=  const=Ncycle_min  OutDataTypeStr=boolean
  NOT(OVP) : Logic  Operator=NOT  IconShape=distinctive  AllPortsSameDT=off  OutDataTypeStr=boolean
  OVC : Logic  IconShape=distinctive  AllPortsSameDT=off  OutDataTypeStr=boolean
  OVC Raw : simulink/Logic and Bit Operations/Compare To Constant  relop=>=  const=Ilimit  OutDataTypeStr=boolean
  OVP : Relay  OnSwitchValue=Vovp  OffSwitchValue=Vovp-10
  Period Done : Scope  Commented=on
      settings: ActiveDisplayYMinimum=-0.12499999999999997  ActiveDisplayYMaximum=1.125  DataLoggingVariableName=ScopeData28
  R : Logic  Operator=OR  IconShape=distinctive  AllPortsSameDT=off  OutDataTypeStr=boolean
  Reset Request : Logic  Operator=OR  Inputs=3  IconShape=distinctive  AllPortsSameDT=off  OutDataTypeStr=boolean
  Restart Ready Protected : Logic  Inputs=4  AllPortsSameDT=off  OutDataTypeStr=boolean
  Restart ready : Scope  Commented=on
      settings: ActiveDisplayYMinimum=-0.12180825947879081  ActiveDisplayYMaximum=1.1472265317427257  DataLoggingVariableName=ScopeData3
  Set : Logic  Inputs=4  AllPortsSameDT=off  OutDataTypeStr=boolean
  Set-Reset Flip-Flop : eeGeneralControl/Set-Reset Flip-Flop  LabelModeActiveChoice=Discrete  UndefState=Reset  Q0=0  Ts=Ts_ctrl
      settings: LibrarySourceBlock=ee_sl_lib/General Control/Set-Reset Flip-Flop
  Startup Pulse : simulink/Logic and Bit Operations/Detect Rise Positive  vinit=0  OutDataTypeStr=boolean
  Step : Step  Time=Tstart  SampleTime=Ts_ctrl
  Step1 : Step  Time=0.21  SampleTime=0
  Ton DONE : RelationalOperator  OutDataTypeStr=boolean  RndMeth=Simplest  InputSameDT=off
  Ton done : Scope  Commented=on
      settings: ActiveDisplayYMinimum=-0.12499999999999997  ActiveDisplayYMaximum=1.125  DataLoggingVariableName=ScopeData16
  ZCD Pulse Limited : simulink/Logic and Bit Operations/Detect Rise Positive  vinit=0  OutDataTypeStr=boolean
  ZCD Valid : Logic  IconShape=distinctive  AllPortsSameDT=off  OutDataTypeStr=boolean
  ZCDpulse limited : Scope  Commented=on
      settings: ActiveDisplayYMinimum=-0.12499999999999997  ActiveDisplayYMaximum=1.125  DataLoggingVariableName=ScopeData13
  ctrl en : Scope  Commented=on
      settings: ActiveDisplayYMinimum=-0.067572366136101847  ActiveDisplayYMaximum=1.141032196932009  DataLoggingVariableName=ScopeData17
  ocp : Scope  Commented=on
      settings: ActiveDisplayYMinimum=-1  ActiveDisplayYMaximum=1  DataLoggingVariableName=ScopeData15
  ovp : Scope  Commented=on
      settings: ActiveDisplayYMinimum=-1  ActiveDisplayYMaximum=1  DataLoggingVariableName=ScopeData14
  GateCmd : Outport
  wires:
  Ton Demand EN Fast/1 -> Restart Ready Protected/1, Set/1
  Restart Ready Protected/1 -> Restart ready/1, ZCD Pulse Limited/1
  GateCmdDelayed/1 -> Data Type Conversion/1, OVC/2, Minimum Cycle Counter/2
  Count One Sample/1 -> Minimum Cycle Counter/1
  Minimum Cycle Counter/1 -> Minimum Period Done/1
  Minimum Period Done/1 -> Period Done/1, Restart Ready Protected/2
  !Ctrl EN/1 -> R/1
  Reset Request/1 -> R/2
  R/1 -> Set-Reset Flip-Flop/2
  Controller EN/1 -> Set/3, ctrl en/1, !Ctrl EN/1  "ControllerEnable"
  Step1/1 -> Controller EN/1
  Set/1 -> Set-Reset Flip-Flop/1
  Ton CMD/1 -> Ton DONE/2
  Ton DONE/1 -> Reset Request/1, Ton done/1
  Elapsed ON/1 -> Ton DONE/1
  !GateCmdDelayed/1 -> Elapsed ON/2, ZCD Valid/2
  Set-Reset Flip-Flop/2 -> !GateCmdDelayed/1
  Gain/1 -> GateCmd/1, Gate CMD/1  "GateCmd"
  Vout/1 -> OVP/1
  Data Type Conversion/1 -> Gain/1, Elapsed ON/1
  Logical Operator/1 -> Set/2
  NOT(OVP)/1 -> Restart Ready Protected/4, Set/4
  ZCD Pulse Limited/1 -> Logical Operator/1, ZCDpulse limited/1
  OVC/1 -> ocp/1, Reset Request/3  "OCP"
  OVC Raw/1 -> OVC/1
  ZCD Valid/1 -> Restart Ready Protected/3  "Zero Ready"
  Current Zero/1 -> ZCD Valid/1
  OVP/1 -> NOT(OVP)/1, Reset Request/2, ovp/1  "OVP"
  Set-Reset Flip-Flop/1 -> GateCmdDelayed/1
  iL/1 -> OVC Raw/1, Current Zero/1
  Step/1 -> Startup Pulse/1
  Startup Pulse/1 -> Logical Operator/2

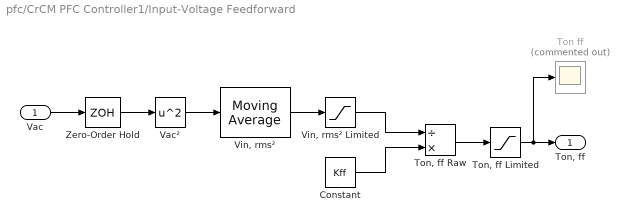
== system pfc/CrCM PFC Controller1/Input-Voltage Feedforward ==
  Vac : Inport
  Constant : Constant  Value=Kff
  Ton ff : Scope  Commented=on
      settings: DataLoggingVariableName=ScopeData29
  "Ton, ff Limited" : Saturate  UpperLimit=Ton_max  LowerLimit=Ton_min
  "Ton, ff Raw" : Product  Inputs=/*
  Vac² : Math  Operator=square
  "Vin, rms²" : eeGeneralControl/Moving Average  VariantControl=Variant1  LabelModeActiveChoice=Discrete  f=Favg  x0=Vin_ff_max^2  BufferSize=8192  Ts=Ts_v
      settings: LibrarySourceBlock=ee_sl_lib/General Control/Moving Average
  "Vin, rms² Limited" : Saturate  UpperLimit=Vin_ff_max^2  LowerLimit=Vin_ff_min^2
  Zero-Order Hold : ZeroOrderHold  SampleTime=Ts_v
  "Ton, ff" : Outport
  wires:
  "Vin, rms² Limited"/1 -> "Ton, ff Raw"/1
  "Vin, rms²"/1 -> "Vin, rms² Limited"/1
  Vac²/1 -> "Vin, rms²"/1
  Zero-Order Hold/1 -> Vac²/1
  Vac/1 -> Zero-Order Hold/1
  Constant/1 -> "Ton, ff Raw"/2
  "Ton, ff Raw"/1 -> "Ton, ff Limited"/1
  "Ton, ff Limited"/1 -> Ton ff/1, "Ton, ff"/1

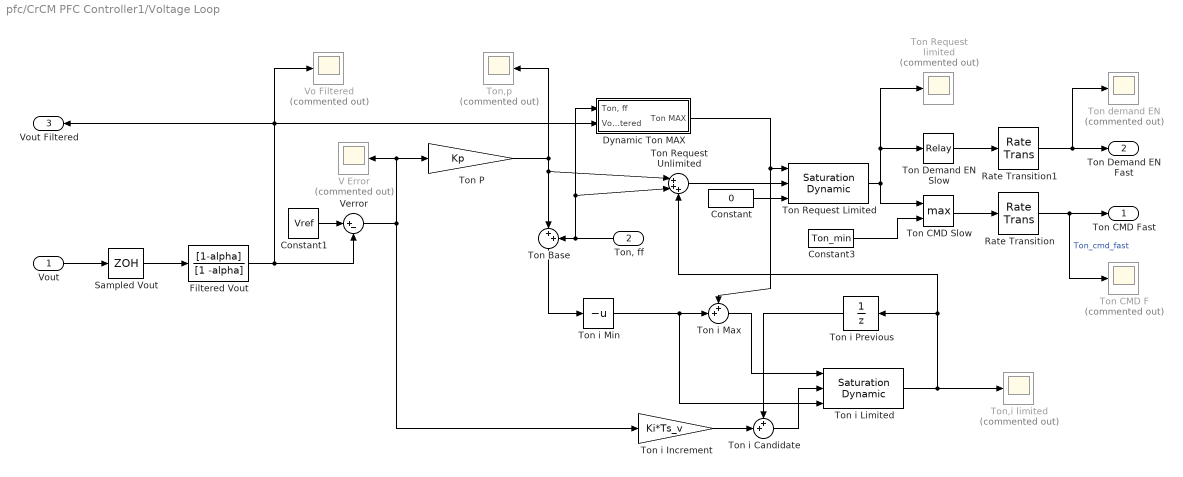
== system pfc/CrCM PFC Controller1/Voltage Loop ==
  Vout : Inport
  "Ton, ff" : Inport  Port=2
  Constant : Constant  Value=0
  Constant1 : Constant  Value=Vref
  Constant3 : Constant  Value=Ton_min
  Dynamic Ton MAX : Subsystem
  Filtered Vout : DiscreteFilter  Numerator=[1-alpha]  Denominator=[1 -alpha]
  Rate Transition : RateTransition  OutPortSampleTime=Ts_ctrl
  Rate Transition1 : RateTransition  OutPortSampleTime=Ts_ctrl
  Sampled Vout : ZeroOrderHold  SampleTime=Ts_v
  Ton Base : Sum  Inputs=|++
  Ton CMD F : Scope  Commented=on
      settings: ActiveDisplayYMinimum=-6.2402343750000437E-7  ActiveDisplayYMaximum=5.61621093750004E-6  DataLoggingVariableName=ScopeData4
  Ton CMD Slow : MinMax  Function=max  Inputs=2
  Ton Demand EN Slow : Relay  OnSwitchValue=0.25e-6  OffSwitchValue=0.15e-6
  Ton P : Gain  Gain=Kp
  Ton Request Limited : simulink/Discontinuities/Saturation Dynamic  OutMin=[]  OutMax=[]  OutDataTypeStr=Inherit: Same as second input  OutDataType=fixdt(1, 16)  OutScaling=2^-10  DoSatur=off
  Ton Request Unlimited : Sum  Inputs=|+++
  Ton Request limited : Scope  Commented=on
      settings: ActiveDisplayYMinimum=-6.2402343750000437E-7  ActiveDisplayYMaximum=5.61621093750004E-6  DataLoggingVariableName=ScopeData31
  Ton demand EN : Scope  Commented=on
      settings: ActiveDisplayYMinimum=-0.12499999999999997  ActiveDisplayYMaximum=1.125  DataLoggingVariableName=ScopeData32
  Ton i Candidate : Sum  Inputs=++|
  Ton i Increment : Gain  Gain=Ki*Ts_v
  Ton i Limited : simulink/Discontinuities/Saturation Dynamic  OutMin=[]  OutMax=[]  OutDataTypeStr=Inherit: Same as second input  OutDataType=fixdt(1, 16)  OutScaling=2^-10  DoSatur=off
  Ton i Max : Sum  Inputs=++|
  Ton i Min : UnaryMinus
  Ton i Previous : UnitDelay  SampleTime=Ts_v  HasFrameUpgradeWarning=on
  Ton,i limited : Scope  Commented=on
      settings: ActiveDisplayYMinimum=-2.1964491979871354E-5  ActiveDisplayYMaximum=-4.8570738523942261E-7  DataLoggingVariableName=ScopeData5
  Ton,p : Scope  Commented=on
      settings: ActiveDisplayYMinimum=-1  ActiveDisplayYMaximum=1  DataLoggingVariableName=ScopeData6
  V Error : Scope  Commented=on
      settings: ActiveDisplayYMinimum=-54.436797901424178  ActiveDisplayYMaximum=450.4929775446027  DataLoggingVariableName=ScopeData12
  Verror : Sum  Inputs=|+-
  Vo Filtered : Scope  Commented=on
      settings: ActiveDisplayYMinimum=-52.339947093671832  ActiveDisplayYMaximum=471.05952384304663  DataLoggingVariableName=ScopeData30
  Ton CMD Fast : Outport
  Ton Demand EN Fast : Outport  Port=2
  Vout Filtered : Outport  Port=3
  wires:
  Rate Transition1/1 -> Ton Demand EN Fast/1, Ton demand EN/1
  Ton Demand EN Slow/1 -> Rate Transition1/1
  Ton CMD Slow/1 -> Rate Transition/1
  Constant3/1 -> Ton CMD Slow/2
  Ton Request Limited/1 -> Ton CMD Slow/1, Ton Demand EN Slow/1, Ton Request limited/1
  Ton i Increment/1 -> Ton i Candidate/2
  Ton i Previous/1 -> Ton i Candidate/1
  Ton i Limited/1 -> Ton Request Unlimited/3, Ton i Previous/1, Ton,i limited/1
  Ton i Candidate/1 -> Ton i Limited/2
  Ton i Min/1 -> Ton i Limited/3, Ton i Max/2
  Ton i Max/1 -> Ton i Limited/1
  Ton Base/1 -> Ton i Min/1
  Dynamic Ton MAX/1(Ton MAX) -> Ton Request Limited/1, Ton i Max/1
  Constant/1 -> Ton Request Limited/3
  "Ton, ff"/1 -> Ton Request Unlimited/2, Dynamic Ton MAX/1("Ton, ff"), Ton Base/2
  Vout/1 -> Sampled Vout/1
  Ton P/1 -> Ton,p/1, Ton Request Unlimited/1, Ton Base/1
  Constant1/1 -> Verror/1
  Sampled Vout/1 -> Filtered Vout/1
  Rate Transition/1 -> Ton CMD F/1, Ton CMD Fast/1  "Ton_cmd_fast"
  Ton Request Unlimited/1 -> Ton Request Limited/2
  Verror/1 -> Ton i Increment/1, Ton P/1, V Error/1
  Filtered Vout/1 -> Vout Filtered/1, Vo Filtered/1, Dynamic Ton MAX/2(Vout Filtered), Verror/2

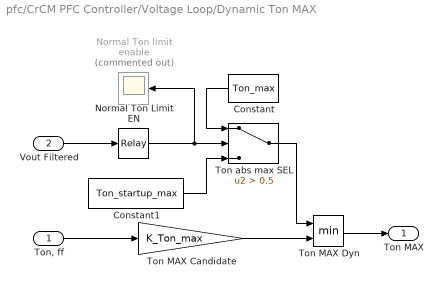
== system pfc/CrCM PFC Controller/Voltage Loop/Dynamic Ton MAX ==
  "Ton, ff" : Inport
  Vout Filtered : Inport  Port=2
  Constant : Constant  Value=Ton_max
  Constant1 : Constant  Value=Ton_startup_max
  Normal Ton Limit EN : Relay  OnSwitchValue=390  OffSwitchValue=370
  Normal Ton limit enable : Scope  Commented=on
      settings: ActiveDisplayYMinimum=-1  ActiveDisplayYMaximum=1  DataLoggingVariableName=ScopeData8
  Ton MAX Candidate : Gain  Gain=K_Ton_max
  Ton MAX Dyn : MinMax  Inputs=2
  Ton abs max SEL : Switch  Criteria=u2 > Threshold  Threshold=0.5  SaturateOnIntegerOverflow=off  InputSameDT=off
  Ton MAX : Outport
  wires:
  Ton MAX Dyn/1 -> Ton MAX/1
  Ton MAX Candidate/1 -> Ton MAX Dyn/2
  "Ton, ff"/1 -> Ton MAX Candidate/1
  Normal Ton Limit EN/1 -> Normal Ton limit enable/1, Ton abs max SEL/2
  Ton abs max SEL/1 -> Ton MAX Dyn/1
  Constant1/1 -> Ton abs max SEL/3
  Constant/1 -> Ton abs max SEL/1
  Vout Filtered/1 -> Normal Ton Limit EN/1

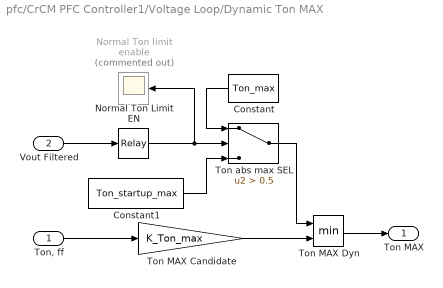
== system pfc/CrCM PFC Controller1/Voltage Loop/Dynamic Ton MAX ==
  "Ton, ff" : Inport
  Vout Filtered : Inport  Port=2
  Constant : Constant  Value=Ton_max
  Constant1 : Constant  Value=Ton_startup_max
  Normal Ton Limit EN : Relay  OnSwitchValue=390  OffSwitchValue=370
  Normal Ton limit enable : Scope  Commented=on
      settings: ActiveDisplayYMinimum=-1  ActiveDisplayYMaximum=1  DataLoggingVariableName=ScopeData8
  Ton MAX Candidate : Gain  Gain=K_Ton_max
  Ton MAX Dyn : MinMax  Inputs=2
  Ton abs max SEL : Switch  Criteria=u2 > Threshold  Threshold=0.5  SaturateOnIntegerOverflow=off  InputSameDT=off
  Ton MAX : Outport
  wires:
  Vout Filtered/1 -> Normal Ton Limit EN/1
  Constant/1 -> Ton abs max SEL/1
  Constant1/1 -> Ton abs max SEL/3
  Ton abs max SEL/1 -> Ton MAX Dyn/1
  Normal Ton Limit EN/1 -> Ton abs max SEL/2, Normal Ton limit enable/1
  "Ton, ff"/1 -> Ton MAX Candidate/1
  Ton MAX Candidate/1 -> Ton MAX Dyn/2
  Ton MAX Dyn/1 -> Ton MAX/1
